simulink model "Model3"  (R2022a)
settings: Solver=VariableStepAuto  StartTime=0.0  StopTime=10.0  RelTol=1e-3  EnableMultiTasking=on
values from neighbouring files (symbols this model uses):
  K1c = Kc(1)    [Exam2018.m]
  K2c = Kc(2)    [Exam2018.m]
  K3c = Kc(3)    [Exam2018.m]
  Nc = K3c    [Exam2018.m]
settings Model: Creator=y.briere  LastModifiedBy=fades
settings SolverCC: AlgebraicLoopSolver=TrustRegion
settings DataIOCC: LimitDataPoints=on  ReturnWorkspaceOutputs=off
settings OptimizationCC: LifeSpan=inf
settings DebuggingCC: UnconnectedInputMsg=warning  UnconnectedOutputMsg=warning  UnconnectedLineMsg=warning  AllowSymbolicDim=off  SFUnexpectedBacktrackingDiag=warning  SFNoUnconditionalDefaultTransitionDiag=warning  SFExecutionAtInitializationDiag=none  SFMachineParentedDataDiag=warning  ArithmeticOperatorsInVariantConditions=warning
settings ModelReferenceCC: PropagateSignalLabelsOutOfModel=off
settings SFSimCC: SimUseLocalCustomCode=off  CustomCodeUndefinedFunction=UseInterfaceOnly
settings RTWCC: RTWUseLocalCustomCode=off
settings CodeAppCC: StateflowObjectComments=on
settings GRTTargetCC: TargetLangStandard=C89/C90 (ANSI)
settings ConfigComp: CovMetricSettings=dw  CovSaveCumulativeToWorkspaceVar=on  CovSaveSingleToWorkspaceVar=on  CovExternalEMLEnable=off

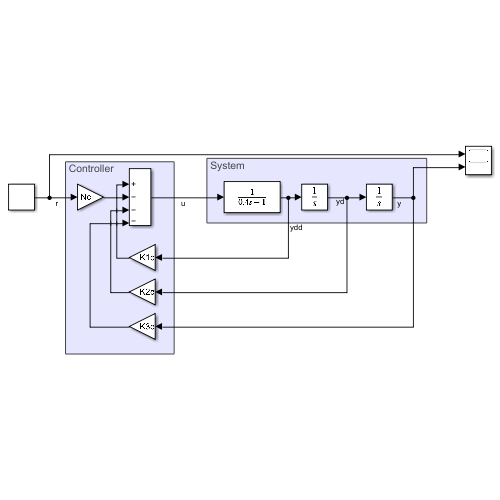
[thumbnail: Simulink's stored preview of the top-level diagram]
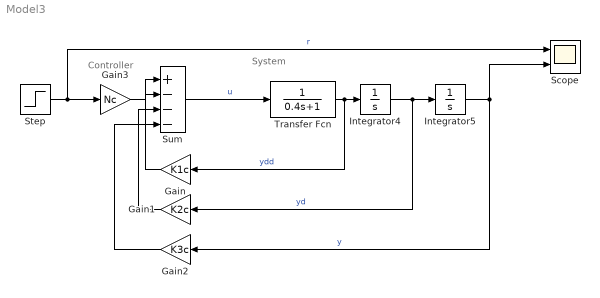
== system Model3 ==
  note: Controller
  note: System
  Gain : Gain  Gain=K1c
  Gain1 : Gain  Gain=K2c
  Gain2 : Gain  Gain=K3c
  Gain3 : Gain  Gain=Nc
  Integrator4 : Integrator
  Integrator5 : Integrator
  Scope : Scope  NumInputPorts=2
  Step : Step  SampleTime=0
  Sum : Sum  Inputs=|+---
  Transfer Fcn : TransferFcn  Denominator=[0.4 1]
  wires:
  Integrator4/1 -> Gain1/1, Integrator5/1  "yd"
  Transfer Fcn/1 -> Gain/1, Integrator4/1  "ydd"
  Sum/1 -> Transfer Fcn/1  "u"
  Integrator5/1 -> Scope/2, Gain2/1  "y"
  Step/1 -> Scope/1, Gain3/1  "r"
  Gain3/1 -> Sum/1
  Gain/1 -> Sum/2
  Gain1/1 -> Sum/3
  Gain2/1 -> Sum/4
